simulink model "ftbf_z_old"  (R2018a)
settings: Solver=VariableStepAuto  StartTime=0.0  StopTime=1  RelTol=1e-3
values from neighbouring files (symbols this model uses):
  a1 = Te/(2*ti)+t1/ti    (= 0.707009440148)    [Trottinette.m]    (also in Trottinette_couple.m)
  dF = dF{1}    [Trottinette.m]    (also in Trottinette_2.m; Trottinette_couple.m; Trottinette_vitesse.m)
  dG = dG{1}    [Trottinette.m]    (also in Trottinette_couple.m)
  E = 0    [Trottinette.m]    (also in Trottinette_couple.m)
  I = 1/ti    (= 344.882653731)    [Trottinette.m]    (also in Trottinette_couple.m)
  nF = nF{1}    [Trottinette.m]    (also in Trottinette_2.m; Trottinette_couple.m; Trottinette_vitesse.m)
  nG = nG{1}    [Trottinette.m]    (also in Trottinette_couple.m)
  Te = 100e-6    (= 0.0001)    [Trottinette.m]    (also in Trottinette_couple.m)
libraries: simulink x1
settings Model: Creator=heusse  LastModifiedBy=cyprienh
settings DataIOCC: ReturnWorkspaceOutputs=on
settings SFSimCC: SimUseLocalCustomCode=on
settings RTWCC: RTWUseLocalCustomCode=on

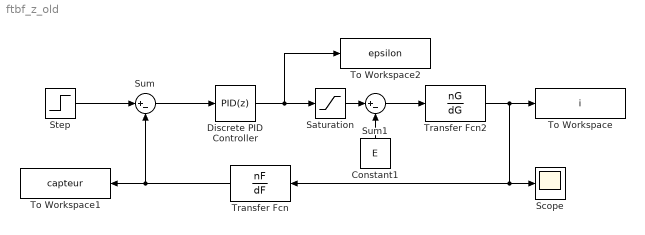
== system ftbf_z_old ==
  Constant1 : Constant  Value=E
  Discrete PID Controller : simulink/Continuous/PID Controller  Controller=PID  TimeDomain=Discrete-time  SampleTime=Te  IntegratorMethod=Forward Euler  FilterMethod=Forward Euler  Form=Parallel  UseFilter=on  ControllerParametersSource=internal  P=a1  I=I  D=0  N=100  InitialConditionSource=internal  InitialConditionForIntegrator=0  InitialConditionForFilter=0  ExternalReset=none  LimitOutput=on  UpperSaturationLimit=0.5  LowerSaturationLimit=-0.5  LinearizeAsGain=off  AntiWindupMode=clamping  Kb=1  TrackingMode=off  Kt=1  PParamMin=[]  PParamMax=[]  IParamMin=[]  IParamMax=[]  DParamMin=[]  DParamMax=[]  NParamMin=[]  NParamMax=[]  KbParamMin=[]  KbParamMax=[]  KtParamMin=[]  KtParamMax=[]  POutMin=[]  POutMax=[]  IOutMin=[]  IOutMax=[]  DOutMin=[]  DOutMax=[]  NOutMin=[]  NOutMax=[]  KbOutMin=[]  KbOutMax=[]  KtOutMin=[]  KtOutMax=[]  IntegratorOutMin=[]  IntegratorOutMax=[]  FilterOutMin=[]  FilterOutMax=[]  SumOutMin=[]  SumOutMax=[]  SumI1OutMin=[]  SumI1OutMax=[]  SumI2OutMin=[]  SumI2OutMax=[]  SumI3OutMin=[]  SumI3OutMax=[]  SumDOutMin=[]  SumDOutMax=[]  SaturationOutMin=[]  SaturationOutMax=[]  IntegratorContinuousStateAttributes=''  IntegratorStateMustResolveToSignalObject=off  IntegratorRTWStateStorageClass=Auto  FilterContinuousStateAttributes=''  FilterStateMustResolveToSignalObject=off  FilterRTWStateStorageClass=Auto  DifferentiatorICPrevScaledInput=0  DifferentiatorOutMin=[]  DifferentiatorOutMax=[]  FilterDiffOutCoefMin=[]  FilterDiffOutCoefMax=[]  SumDenOutMin=[]  SumDenOutMax=[]  SumNumOutMin=[]  SumNumOutMax=[]  ReciprocalOutMin=[]  ReciprocalOutMax=[]  DivideOutMin=[]  DivideOutMax=[]  TunerSelectOption=Transfer Function Based (PID Tuner App)
  Saturation : Saturate
  Scope : Scope
  Step : Step  Time=0  After=1.65  SampleTime=0
  Sum : Sum  Inputs=|+-
  Sum1 : Sum  Inputs=|+-
  To Workspace : ToWorkspace  VariableName=i  SaveFormat=Timeseries  SampleTime=-1
  To Workspace1 : ToWorkspace  VariableName=capteur  SaveFormat=Timeseries  SampleTime=-1
  To Workspace2 : ToWorkspace  VariableName=epsilon  SaveFormat=Timeseries  SampleTime=-1
  Transfer Fcn : TransferFcn  Numerator=nF  Denominator=dF
  Transfer Fcn2 : TransferFcn  Numerator=nG  Denominator=dG
  wires:
  Step/1 -> Sum/1
  Sum/1 -> Discrete PID Controller/1
  Sum1/1 -> Transfer Fcn2/1
  Discrete PID Controller/1 -> Saturation/1, To Workspace2/1
  Transfer Fcn2/1 -> To Workspace/1, Transfer Fcn/1, Scope/1
  Constant1/1 -> Sum1/2
  Saturation/1 -> Sum1/1
  Transfer Fcn/1 -> Sum/2, To Workspace1/1
